simulink model "problem1_pv"  (R2023b)
settings: Solver=ode1  StartTime=0  StopTime=9  FixedStep=1/2880000  RelTol=1e-3
libraries: spsSeriesRLCBranchLib x7, spsMeanLib x3, spsDiodeLib x2, spsIGBTDiodeLib x2, spsMultimeterLib x2, spsPWMGeneratorDCDCLib x2, spsCurrentMeasurementLib x1, spsDCVoltageSourceLib x1, slpidlib x1, spsPVArrayLib x1, spsSawtoothGeneratorLib x1, SignalEditorBlockLib x1
settings Model: Creator=lmanglicmot  LastModifiedBy=lmanglicmot

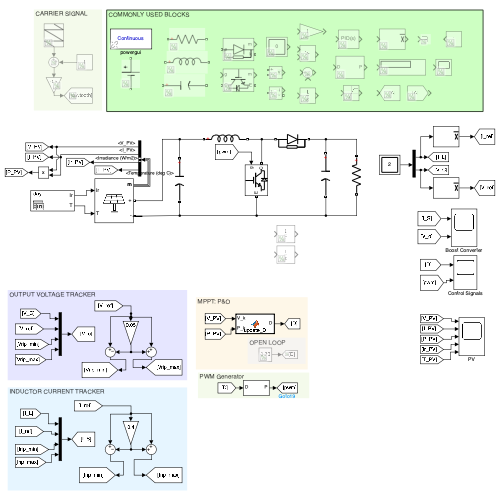
[thumbnail: Simulink's stored preview of the top-level diagram]
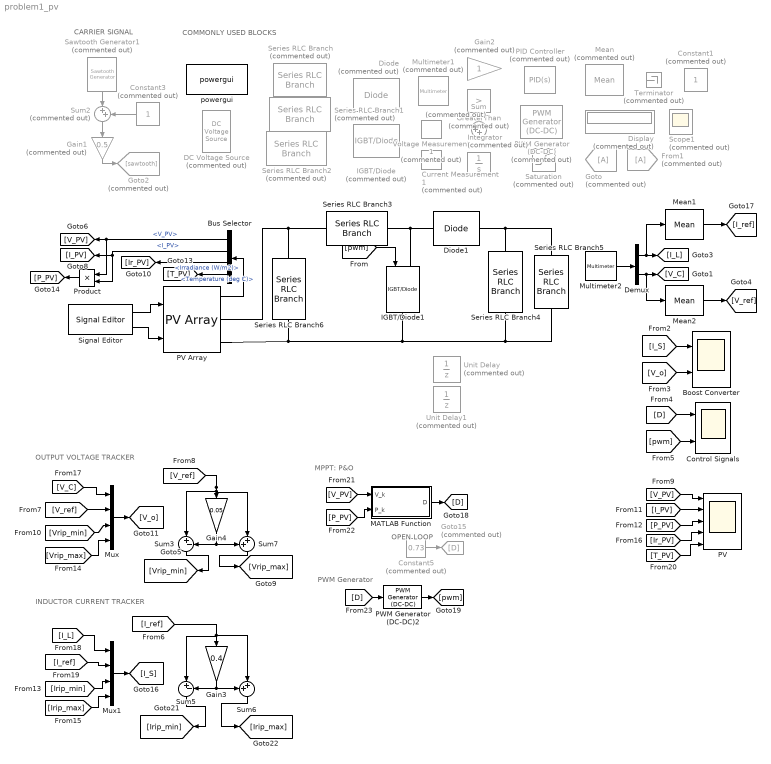
== system problem1_pv ==
  note: CARRIER SIGNAL
  note: COMMONLY USED BLOCKS
  note: OUTPUT VOLTAGE TRACKER
  note: INDUCTOR CURRENT TRACKER
  note: OPEN LOOP
  note: MPPT: P&O
  note: PWM Generator
  Boost Converter : Scope  NumInputPorts=2
  Bus Selector : BusSelector  OutputSignals=V_PV,I_PV,Irradiance (W/m2),Temperature (deg C)
  Constant1 : Constant  Commented=on
  Constant3 : Constant  Commented=on
  Constant5 : Constant  Commented=on  Value=0.73
  Control Signals : Scope  NumInputPorts=2
  Current Measurement1 : spsCurrentMeasurementLib/Current Measurement  Commented=on  PhasorSimulation=off  OutputType=Complex  PSBequivalent=0
  DC Voltage Source : spsDCVoltageSourceLib/DC Voltage Source  Commented=on  Amplitude=100  Measurements=None
  Demux : Demux  Outputs=2
  Diode : spsDiodeLib/Diode  Commented=on  Ron=0.001  Lon=0  Vf=0.8  IC=0  UseSnubber=0  Rs=500  Cs=250e-9  Measurements=on
  Diode1 : spsDiodeLib/Diode  Ron=0.001  Lon=0  Vf=0.8  IC=0  UseSnubber=0  Rs=500  Cs=250e-9  Measurements=off
  Display : Display  Commented=on
  From1 : From  Commented=on
  Gain1 : Gain  Commented=on  Gain=0.5
  Gain2 : Gain  Commented=on
  Gain3 : Gain  Gain=0.4
  Gain4 : Gain  Gain=0.05
  Goto : Goto  Commented=on
  Goto15 : Goto  Commented=on  GotoTag=D
  Goto2 : Goto  Commented=on  GotoTag=sawtooth
  GreaterThan : RelationalOperator  Commented=on  Operator=>  OutDataTypeStr=boolean  RndMeth=Simplest  InputSameDT=off
  IGBT/Diode : spsIGBTDiodeLib/IGBT//Diode  Commented=on  Ron=1e-3  Rs=1e5  Cs=inf  Measurements=on
  IGBT/Diode1 : spsIGBTDiodeLib/IGBT//Diode  Ron=1e-3  Rs=1e5  Cs=inf  Measurements=off
  Integrator : Integrator  Commented=on
  MATLAB Function : MATLAB Function  TreatAsAtomicUnit=on
  Mean : spsMeanLib/Mean  Commented=on  Freq=60  Vinit=0  Ts=0
  Mean1 : spsMeanLib/Mean  Freq=60  Vinit=0  Ts=0
  Mean2 : spsMeanLib/Mean  Freq=60  Vinit=0  Ts=0
  Multimeter1 : spsMultimeterLib/Multimeter  Commented=on  L=1  sel=1  yselected={}  Gain=0  OutputType=Complex  PlotAtSimulationStop=off  PhasorSimulation=off
  Multimeter2 : spsMultimeterLib/Multimeter  L=3  sel=[3 1]  yselected={}  Gain=[1 1]  OutputType=Complex  PlotAtSimulationStop=off  PhasorSimulation=off
  Mux : Mux
  Mux1 : Mux
  PID Controller : slpidlib/PID Controller  Commented=on  Controller=PID  Form=Parallel  TimeDomain=Continuous-time  UseExternalTs=off  SampleTime=-1  IntegratorMethod=Forward Euler  FilterMethod=Forward Euler  ControllerParametersSource=internal  P=1  I=1  UseKiTs=off  D=0  N=100  UseFilter=on  TunerSelectOption=Transfer Function Based (PID Tuner App)  InitialConditionSource=internal  InitialConditionForIntegrator=0  InitialConditionForFilter=0  DifferentiatorICPrevScaledInput=0  ExternalReset=none  TrackingMode=off  Kt=1  LimitOutput=off  SatLimitsSource=internal  UpperSaturationLimit=inf  LowerSaturationLimit=-inf  LinearizeAsGain=on  AntiWindupMode=none  Kb=1  LimitIntegrator=off  UpperIntegratorSaturationLimit=inf  LowerIntegratorSaturationLimit=-inf  POutMin=[]  POutMax=[]  IOutMin=[]  IOutMax=[]  DOutMin=[]  DOutMax=[]  NOutMin=[]  NOutMax=[]  SumOutMin=[]  SumOutMax=[]  SaturationOutMin=[]  SaturationOutMax=[]  PParamMin=[]  PParamMax=[]  IParamMin=[]  IParamMax=[]  DParamMin=[]  DParamMax=[]  NParamMin=[]  NParamMax=[]  KbParamMin=[]  KbParamMax=[]  KtParamMin=[]  KtParamMax=[]  KbOutMin=[]  KbOutMax=[]  KtOutMin=[]  KtOutMax=[]  IntegratorOutMin=[]  IntegratorOutMax=[]  FilterOutMin=[]  FilterOutMax=[]  SumI1OutMin=[]  SumI1OutMax=[]  SumI2OutMin=[]  SumI2OutMax=[]  SumI3OutMin=[]  SumI3OutMax=[]  SumI4OutMin=[]  SumI4OutMax=[]  SumDOutMin=[]  SumDOutMax=[]  DifferentiatorOutMin=[]  DifferentiatorOutMax=[]  FilterDiffOutCoefMin=[]  FilterDiffOutCoefMax=[]  ReciprocalOutMin=[]  ReciprocalOutMax=[]  SumDenOutMin=[]  SumDenOutMax=[]  SumNumOutMin=[]  SumNumOutMax=[]  DivideOutMin=[]  DivideOutMax=[]  UdiffTsProdOutMin=[]  UdiffTsProdOutMax=[]  NTsProdOutMin=[]  NTsProdOutMax=[]  UintegralTsProdOutMin=[]  UintegralTsProdOutMax=[]  UngainTsProdOutMin=[]  UngainTsProdOutMax=[]  ClampingZeroOutDataTypeStr=Inherit: Inherit via back propagation  ClampingZeroOutMin=[]  ClampingZeroOutMax=[]  FilterDenConstantOutDataTypeStr=Inherit: Inherit via back propagation  FilterDenConstantOutMin=[]  FilterDenConstantOutMax=[]  PCopyOutDataTypeStr=Inherit: Inherit via back propagation  PCopyOutMin=[]  PCopyOutMax=[]  NCopyOutDataTypeStr=Inherit: Inherit via back propagation  NCopyOutMin=[]  NCopyOutMax=[]  IntegratorContinuousStateAttributes=''  IntegratorStateMustResolveToSignalObject=off  IntegratorRTWStateStorageClass=Auto  FilterContinuousStateAttributes=''  FilterStateMustResolveToSignalObject=off  FilterRTWStateStorageClass=Auto  ParallelPVariant=InternalParameters  IdealPVariant=Disabled  IVariant=InternalParameters  DVariant=InternalParameters  IntegratorVariant=Continuous  SatVariant=Disabled  AWVariant=Passthrough  PCopyVariant=Disabled  TRVariant=Disabled  FdbkBlocksVariant=Forward  IdealPFdbkVariant=Disabled  SatFdbkVariant=Disabled  DerivativeFilterVariant=ContFilter  NVariant=InternalParameters  NCopyVariant=Disabled  FilterICVariant=InternalICsFilter  IntegratorICVariant=InternalICs  ExternalResetVariant=Disabled  TRSumVariant=Passthrough  SumFdbkVariant=Disabled  SumVariant=Sum_PID  TsampFilterVariant=InternalTs  TsampNgainVariant=Passthrough  TsampIntegralVariant=Disabled_SignalSpec  ExternalSaturationOutDataTypeStr=Inherit: Same as second input
  PV : Scope  NumInputPorts=5
  PV Array : spsPVArrayLib/PV Array  Npar=10  Nser=5  PlotType=array @ 1000 W/m2 & specified temperatures  S_vec="[ 1000  500  100 ]"  Temp_C_vec="[ 45 25  ]"  ModuleName=Solaria Corporation Solaria 280  PlotWhenSelected=off  Pm=280.176  Ncell=72  Voc=44.57  Isc=8.27  Vm=35.92  Im=7.8  beta_Voc_pc=-0.33  alpha_Isc_pc=0.05  beta_Voc=-0.14708  alpha_Isc=0.004135  IL=8.2768  I0=9.3071e-11  nI=0.95598  Rsh=699.2081  Rs=0.43576  RobustModel=off  RobustCellTemperature=313.3991  BAL=on  Tc=1e-6  Tfilter=5e-5
  PWM Generator (DC-DC) : spsPWMGeneratorDCDCLib/PWM Generator (DC-DC)  Commented=on  Fsw=5000  Ts=0
  PWM Generator (DC-DC)2 : spsPWMGeneratorDCDCLib/PWM Generator (DC-DC)  Fsw=12e3  Ts=0
  Product : Product
  Saturation : Saturate  Commented=on
  Sawtooth Generator1 : spsSawtoothGeneratorLib/Sawtooth Generator  Commented=on  Freq=12e3  Phase=180  Ts=0
  Scope1 : Scope  Commented=on
  Series RLC Branch : spsSeriesRLCBranchLib/Series RLC Branch  Commented=on  LConnTagsString=__new0  RConnTagsString=__new0  BranchType=R  Resistance=1  Inductance=1e-3  SetiL0=off  InitialCurrent=0  Capacitance=1e-6  Setx0=off  InitialVoltage=0  Measurements=None
  Series RLC Branch1 : spsSeriesRLCBranchLib/Series RLC Branch  Commented=on  LConnTagsString=__new0  RConnTagsString=__new0  BranchType=L  Resistance=1  Inductance=1e-3  SetiL0=off  InitialCurrent=0  Capacitance=1e-6  Setx0=off  InitialVoltage=0  Measurements=None
  Series RLC Branch2 : spsSeriesRLCBranchLib/Series RLC Branch  Commented=on  LConnTagsString=__new0  RConnTagsString=__new0  BranchType=C  Resistance=1  Inductance=1e-3  SetiL0=off  InitialCurrent=0  Capacitance=1e-6  Setx0=off  InitialVoltage=0  Measurements=None
  Series RLC Branch3 : spsSeriesRLCBranchLib/Series RLC Branch  LConnTagsString=__new0  RConnTagsString=__new0  BranchType=L  Resistance=1  Inductance=2e-2  SetiL0=off  InitialCurrent=0  Capacitance=1e-6  Setx0=off  InitialVoltage=0  Measurements=Branch current
  Series RLC Branch4 : spsSeriesRLCBranchLib/Series RLC Branch  LConnTagsString=__new0  RConnTagsString=__new0  BranchType=C  Resistance=1  Inductance=1e-3  SetiL0=off  InitialCurrent=0  Capacitance=3.6e-3  Setx0=off  InitialVoltage=0  Measurements=Branch voltage
  Series RLC Branch5 : spsSeriesRLCBranchLib/Series RLC Branch  LConnTagsString=__new0  RConnTagsString=__new0  BranchType=R  Resistance=20  Inductance=1e-3  SetiL0=off  InitialCurrent=0  Capacitance=1e-6  Setx0=off  InitialVoltage=0  Measurements=None
  Series RLC Branch6 : spsSeriesRLCBranchLib/Series RLC Branch  LConnTagsString=__new0  RConnTagsString=__new0  BranchType=C  Resistance=1  Inductance=1e-3  SetiL0=off  InitialCurrent=0  Capacitance=1200e-6  Setx0=off  InitialVoltage=0  Measurements=Branch voltage
  Signal Editor : SignalEditorBlockLib/Signal Editor  FileName=irradiance.mat  ActiveScenario=day  ActiveSignal=Ir  IsBus=off  OutputBusObjectStr=Bus: BusObject  SampleTime=0  Interpolate=off  ZeroCross=off  OutputAfterFinalValue=Setting to zero  Unit=inherit  PreserveSignalName=on  ApplySigPropsToAllScenarios=on  ApplySigPropsToAllSignals=off
  Sum : Sum  Commented=on  Inputs=|++
  Sum2 : Sum  Commented=on  Inputs=|++
  Sum3 : Sum  Inputs=|+-
  Sum5 : Sum  Inputs=|+-
  Sum6 : Sum  Inputs=++|
  Sum7 : Sum  Inputs=++|
  Terminator : Terminator  Commented=on
  Unit Delay : UnitDelay  Commented=on  SampleTime=-1  HasFrameUpgradeWarning=on
  Unit Delay1 : UnitDelay  Commented=on  SampleTime=-1  HasFrameUpgradeWarning=on
  Voltage Measurement1 : spsVoltageMeasurementLib/Voltage Measurement  Commented=on  PhasorSimulation=off  OutputType=Complex  PSBequivalent=0
  powergui : sps_lib/powergui  Priority=1  SimulationMode=Continuous  SampleTime=1/20000  frequency=60  Iterations=50  frequencyindice=0  Pbase=100e6  ErrMax=1e-4  UnitsV=kV  UnitsW=MW  buscounter=0  FunctionMessages=off  echomessages=off  EnableUseOfTLC=off  CurrentSourceSwitches=off  DisableSnubberDevices=off  DisableRonSwitches=off  DisableVfSwitches=off  DisplayEquations=off  AutomaticDiscreteSolvers=off  SolverType=Tustin/Backward Euler (TBE)  Interpol=off  ExternalGateDelay=off  methode=off  Ts=100  x0status=blocks  SPID=on  SwTol=0  HookPort=off  NonlinearTolerance=1e-4  nMaxIteration=100  ContinueOnMaxIteration=off  RestoreLinks=warning  ResistiveCurrentMeasurement=off  Frange=[0:2:500]  Ylog=off  Xlog=on  ShowGrid=off  save=off  variable=ZData  structure=0  ZoomFFT=off  StartTime=0.0  cycles=1  DisplayStyle=1  fundamental=60  FreqAxis=off  MaxFrequency=1000  frequencyindicesteady=1  RmsSteady=1  display=off
  wires:
  Sum2/1 -> Gain1/1
  Constant3/1 -> Sum2/2
  Sawtooth Generator1/1 -> Sum2/1
  Gain1/1 -> Goto2/1
  Gain4/1 -> Sum3/2, Sum7/1
  Sum7/1 -> [Vrip_max]
  Sum3/1 -> [Vrip_min]
  Mux/1 -> [V_o]
  [V_C] -> Mux/1
  [V_ref] -> Mux/2
  [V_ref] -> Sum7/2, Sum3/1, Gain4/1
  [Vrip_min] -> Mux/3
  [Vrip_max] -> Mux/4
  [pwm] -> IGBT/Diode1/1
  Multimeter2/1 -> Demux/1
  [I_ref] -> Sum6/2, Sum5/1, Gain3/1
  [Irip_max] -> Mux1/4
  Gain3/1 -> Sum5/2, Sum6/1
  [I_L] -> Mux1/1
  Sum6/1 -> [Irip_max]
  Sum5/1 -> [Irip_min]
  [Irip_min] -> Mux1/3
  [I_ref] -> Mux1/2
  Mux1/1 -> [I_S]
  [I_S] -> Boost Converter/1
  Demux/1 -> Mean1/1, [I_L]
  Demux/2 -> Mean2/1, [V_C]
  [V_o] -> Boost Converter/2
  [D] -> Control Signals/1
  [pwm] -> Control Signals/2
  Mean1/1 -> [I_ref]
  Signal Editor/1 -> PV Array/1
  Mean2/1 -> [V_ref]
  PV Array/1 -> Bus Selector/1
  Bus Selector/1 -> Product/1, [V_PV]  "<V_PV>"
  Bus Selector/2 -> [I_PV], Product/2  "<I_PV>"
  Bus Selector/3 -> [Ir_PV]  "<Irradiance (W/m2)>"
  Bus Selector/4 -> [T_PV]  "<Temperature (deg C)>"
  Product/1 -> [P_PV]
  [V_PV] -> PV/1
  [I_PV] -> PV/2
  [P_PV] -> PV/3
  [Ir_PV] -> PV/4
  [T_PV] -> PV/5
  Signal Editor/2 -> PV Array/2
  MATLAB Function/1(D) -> [D]
  Constant5/1 -> Goto15/1
  [V_PV] -> MATLAB Function/1(V_k)
  [P_PV] -> MATLAB Function/2(P_k)
  [D] -> PWM Generator (DC-DC)2/1
  PWM Generator (DC-DC)2/1 -> [pwm]
  connections:
  Diode1/LConn1 -- IGBT/Diode1/LConn1 -- Series RLC Branch3/RConn1
  Series RLC Branch4/LConn1 -- Series RLC Branch5/LConn1 -- Diode1/RConn1
  PV Array/RConn1 -- Series RLC Branch3/LConn1 -- Series RLC Branch6/LConn1
  PV Array/RConn2 -- Series RLC Branch5/RConn1 -- Series RLC Branch4/RConn1 -- IGBT/Diode1/RConn1 -- Series RLC Branch6/RConn1

== matlab function problem1_pv/MATLAB Function ==
  settings: updateMethod=DISCRETE
  data: V_k input; D output; P_k input
function D = update_D(V_k, P_k)

persistent  P_k_1 V_k_1  D_k_1 temp step_size

step_size = 0.01;
D_init = 0;       % initialize D near 0.733 to step up from 80V to 300 V
D_min = 0;
D_max = 0.9;

if isempty(V_k_1)
    V_k_1 = 0;
    P_k_1 = 0;
    D_k_1 = D_init;
end 

dV = V_k - V_k_1;
dP = P_k - P_k_1;

if dP ~= 0 && V_k > 50
    if dP < 0
        if dV < 0
            temp = D_k_1 - step_size;
        else 
            temp = D_k_1 + step_size;
        end
    else
        if dV < 0
            temp = D_k_1 + step_size;
        else
            temp = D_k_1 - step_size;
        end
    end
else
    temp = D_k_1;
end

if temp > D_max
    temp = D_max;
elseif temp < D_min
    temp = D_min;
end

D_k_1 = temp;
P_k_1 = P_k;
V_k_1 = V_k;
D = temp;
